simulink model "quick_release_expt_model_hg"  (R2024b)
settings: Solver=VariableStepAuto  StartTime=0.0  StopTime=2  MaxStep=1e-3  RelTol=1e-6  AbsTol=1e-6
values from neighbouring files (symbols this model uses):
  c = log(0.05)    [hill_type_muscle_params_hg.m]
  e_ref_see = 0.04    [hill_type_muscle_params_hg.m]
  F_max = 6000    [hill_type_muscle_params_hg.m]
  g = 9.81    [hill_type_muscle_params_hg.m]
  K = 5    [hill_type_muscle_params_hg.m]
  l_opt = 0.1    [hill_type_muscle_params_hg.m]
  l_ref_mtc = 0.5    [hill_type_muscle_params_hg.m]
  l_rest = 0.4    [hill_type_muscle_params_hg.m]
  m = 450    [hill_type_muscle_params_hg.m]
  N = 1.5    [hill_type_muscle_params_hg.m]
  tau = 0.01    [hill_type_muscle_params_hg.m]
  v_max = 12 * l_opt    (= 1.2)    [hill_type_muscle_params_hg.m]
  w = 0.4    [hill_type_muscle_params_hg.m]
settings Model: Creator=athar  LastModifiedBy=athar
settings SolverCC: AutoScaleAbsTol=off

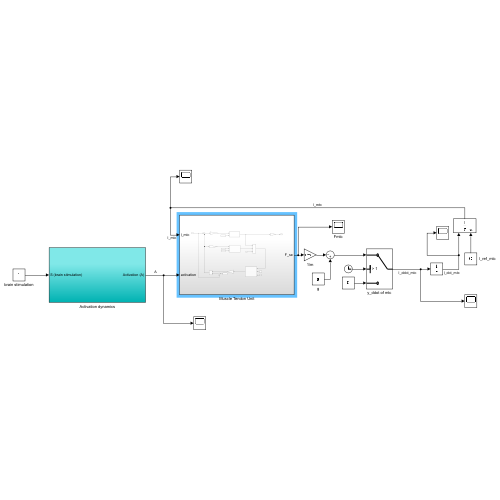
[thumbnail: Simulink's stored preview of the top-level diagram]
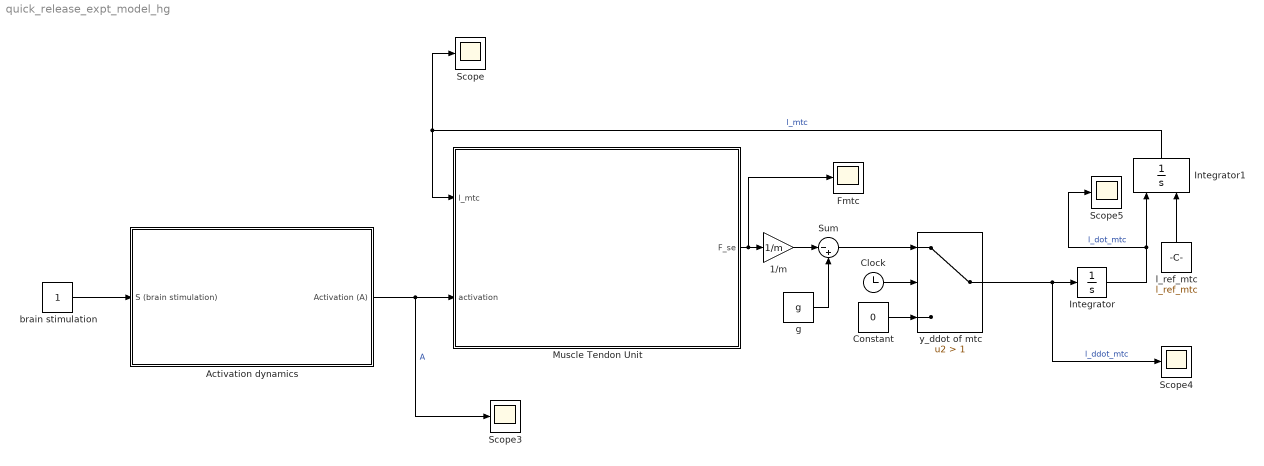
== system quick_release_expt_model_hg ==
  1/m : Gain  Gain=1/m
  Activation dynamics : Subsystem
  Clock : Clock
  Constant : Constant  Value=0
  Fmtc : Scope
  Integrator : Integrator
  Integrator1 : Integrator  InitialConditionSource=external
  Muscle Tendon Unit : Subsystem
  Scope{,3..5} (4 alike) : Scope
  Sum : Sum  Inputs=|-+
  brain stimulation : Constant
  g : Constant  Value=g
  l_ref_mtc : Constant  Value=l_ref_mtc
  y_ddot of mtc : Switch  Criteria=u2 > Threshold  Threshold=1  SaturateOnIntegerOverflow=off  InputSameDT=off
  wires:
  brain stimulation/1 -> Activation dynamics/1(S (brain stimulation))
  Activation dynamics/1(Activation (A)) -> Scope3/1, Muscle Tendon Unit/2(activation)  "A"
  Muscle Tendon Unit/1(F_se) -> Fmtc/1, 1/m/1
  Constant/1 -> y_ddot of mtc/3
  g/1 -> Sum/2
  1/m/1 -> Sum/1
  Sum/1 -> y_ddot of mtc/1
  Clock/1 -> y_ddot of mtc/2
  y_ddot of mtc/1 -> Scope4/1, Integrator/1  "l_ddot_mtc"
  Integrator/1 -> Scope5/1, Integrator1/1  "l_dot_mtc"
  l_ref_mtc/1 -> Integrator1/2
  Integrator1/1 -> Scope/1, Muscle Tendon Unit/1(l_mtc)  "l_mtc"

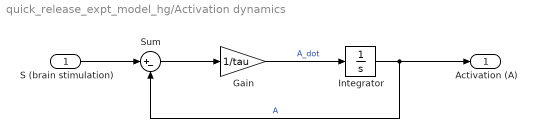
== system quick_release_expt_model_hg/Activation dynamics ==
  S (brain stimulation) : Inport
  Gain : Gain  Gain=1/tau
  Integrator : Integrator  InitialCondition=0.01
  Sum : Sum  Inputs=|+-
  Activation (A) : Outport
  wires:
  S (brain stimulation)/1 -> Sum/1
  Sum/1 -> Gain/1
  Gain/1 -> Integrator/1  "A_dot"
  Integrator/1 -> Sum/2, Activation (A)/1  "A"

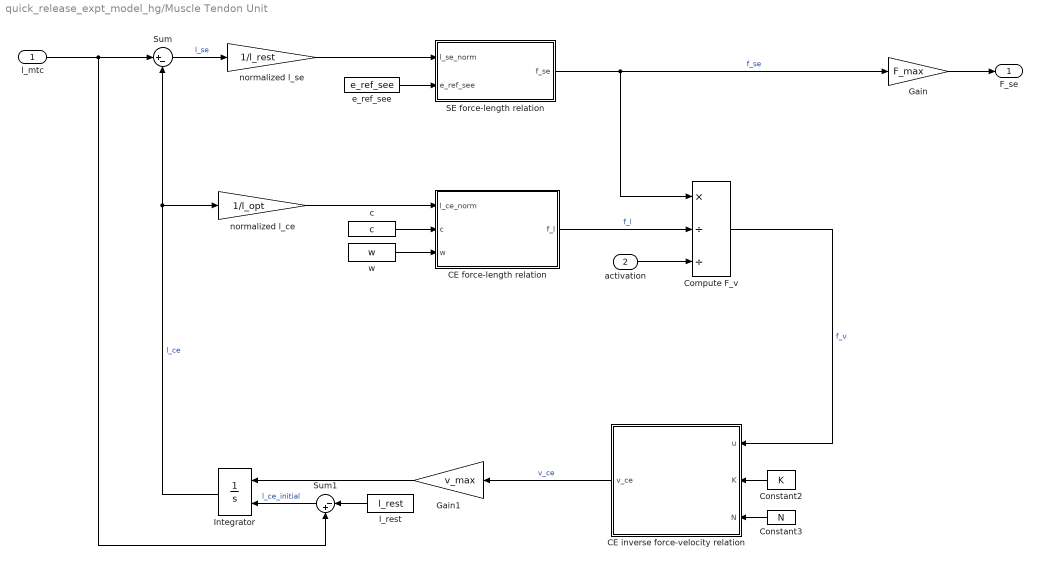
== system quick_release_expt_model_hg/Muscle Tendon Unit ==
  l_mtc : Inport
  activation : Inport  Port=2
  CE force-length relation : MATLAB Function  TreatAsAtomicUnit=on
  CE inverse force-velocity relation : MATLAB Function  TreatAsAtomicUnit=on
  Compute F_v : Product  Inputs=*//
  Constant2 : Constant  Value=K
  Constant3 : Constant  Value=N
  Gain : Gain  Gain=F_max
  Gain1 : Gain  Gain=v_max
  Integrator : Integrator  InitialConditionSource=external
  SE force-length relation : MATLAB Function  TreatAsAtomicUnit=on
  Sum : Sum  Inputs=|+-
  Sum1 : Sum  Inputs=|-+
  c : Constant  Value=c
  e_ref_see : Constant  Value=e_ref_see
  l_rest : Constant  Value=l_rest
  normalized l_ce : Gain  Gain=1/l_opt
  normalized l_se : Gain  Gain=1/l_rest
  w : Constant  Value=w
  F_se : Outport
  wires:
  CE force-length relation/1(f_l) -> Compute F_v/2  "f_l"
  SE force-length relation/1(f_se) -> Compute F_v/1, Gain/1  "f_se"
  Integrator/1 -> normalized l_ce/1, Sum/2  "l_ce"
  activation/1 -> Compute F_v/3
  CE inverse force-velocity relation/1(v_ce) -> Gain1/1  "v_ce"
  Sum/1 -> normalized l_se/1  "l_se"
  c/1 -> CE force-length relation/2(c)
  Compute F_v/1 -> CE inverse force-velocity relation/1(u)  "f_v"
  e_ref_see/1 -> SE force-length relation/2(e_ref_see)
  Sum1/1 -> Integrator/2  "l_ce_initial"
  Constant2/1 -> CE inverse force-velocity relation/2(K)
  l_mtc/1 -> Sum1/2, Sum/1
  Constant3/1 -> CE inverse force-velocity relation/3(N)
  w/1 -> CE force-length relation/3(w)
  normalized l_se/1 -> SE force-length relation/1(l_se_norm)
  normalized l_ce/1 -> CE force-length relation/1(l_ce_norm)
  Gain/1 -> F_se/1
  Gain1/1 -> Integrator/1
  l_rest/1 -> Sum1/1

== matlab function quick_release_expt_model_hg/Muscle Tendon Unit/SE force-length relation ==
  data: l_se_norm input; f_se output; e_ref_see input
function f_se = f_se(l_se_norm, e_ref_see)

e = l_se_norm - 1;

if e > 0
    f_se = (e / e_ref_see)^2;
else
    f_se = 0;
end

== matlab function quick_release_expt_model_hg/Muscle Tendon Unit/CE inverse force-velocity relation ==
  data: u input; v_ce output; K input; N input
function v_ce = f_v_inverse(u, K, N)
  
    if u < 1
        v_ce = (u - 1)/(1 + K * u);
    
    elseif (1 <= u) && (u < N)
        v_ce = (1 - u) / ((1 - N) + 7.56 * K * (u - N));
    
    elseif u >= N
        v_ce = 1;
    
    else 
        v_ce = 0;
    end
    
end

== matlab function quick_release_expt_model_hg/Muscle Tendon Unit/CE force-length relation ==
  data: l_ce_norm input; f_l output; c input; w input
function f_l = f_l(l_ce_norm, c , w)

    f_l = exp(c * (abs((l_ce_norm - 1) / w)^3));

end
